simulink model "local_observer_prec"  (R2024b)
settings: Solver=VariableStepAuto  StartTime=0.0  StopTime=20.0  RelTol=1e-3
values from neighbouring files (symbols this model uses):
  A = [0 1; 880.87 0]    [Project.m]    (also in debug_simulink_integration.m; project_multiple_run.m; project_single_run.m)
  B = [0; -9.9453]    [Project.m]    (also in debug_simulink_integration.m; find_hurwitz_F.m = c * eye(n); project_multiple_run.m; project_single_run.m)
  C = [708.27 0]    [Project.m]    (also in debug_simulink_integration.m; project_multiple_run.m; project_single_run.m)
  c = cmin * 2    [Project.m]    (also in project_multiple_run.m = cmin * c_weights(ic); project_single_run.m = cmin)
  K = R^(-1) * B' *Pc    [Project.m]    (also in find_hurwitz_F.m = lqr(A, B, Q, R); project_multiple_run.m = R^(-1) * B' * Pc; project_single_run.m = R^(-1) * B' * Pc)
undefined symbols (not defined in the file or in its folder): A_adj, G_pinning, K_place
settings Model: Creator=fvero  LastModifiedBy=fabio
settings ConfigComp: CovBoundaryAbsTol=1.0e-5

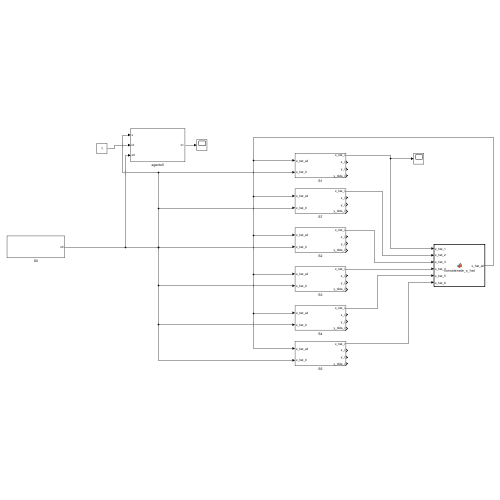
[thumbnail: Simulink's stored preview of the top-level diagram]
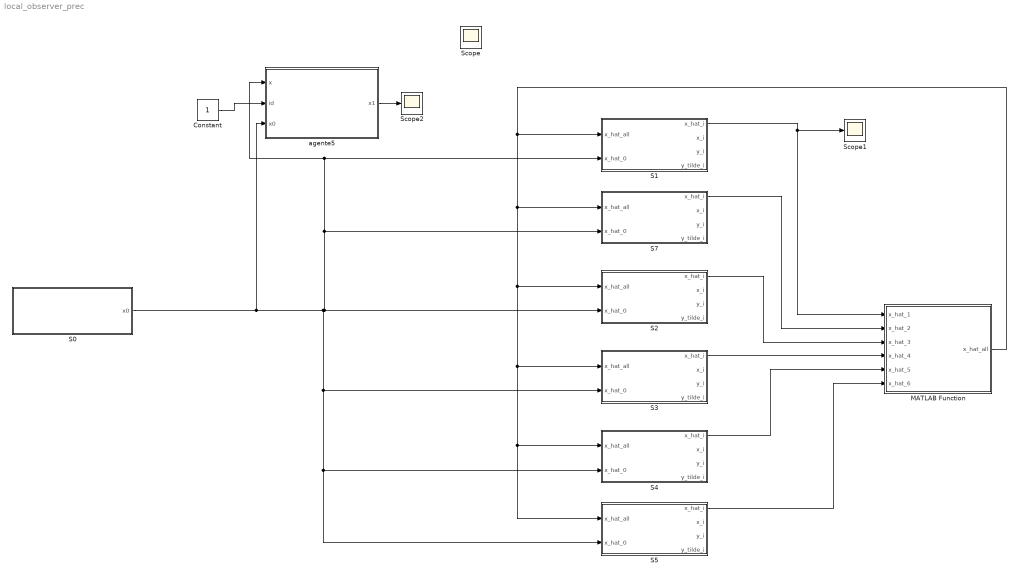
== system local_observer_prec ==
  Constant : Constant
  MATLAB Function : MATLAB Function  TreatAsAtomicUnit=on
  S0 : Subsystem
  S1 : Subsystem
  S2 : Subsystem
  S3 : Subsystem
  S4 : Subsystem
  S5 : Subsystem
  S7 : Subsystem
  Scope1 : Scope
  Scope2 : Scope
  agente5 : Subsystem
  Scope : Scope
  wires:
  S1/1(x_hat_i) -> Scope1/1, MATLAB Function/1(x_hat_1)
  S7/1(x_hat_i) -> MATLAB Function/2(x_hat_2)
  S2/1(x_hat_i) -> MATLAB Function/3(x_hat_3)
  S3/1(x_hat_i) -> MATLAB Function/4(x_hat_4)
  S4/1(x_hat_i) -> MATLAB Function/5(x_hat_5)
  S5/1(x_hat_i) -> MATLAB Function/6(x_hat_6)
  MATLAB Function/1(x_hat_all) -> S7/1(x_hat_all), S2/1(x_hat_all), S3/1(x_hat_all), S5/1(x_hat_all), S4/1(x_hat_all), S1/1(x_hat_all)
  S0/1(x0) -> agente5/3(x0), S3/2(x_hat_0), S5/2(x_hat_0), S4/2(x_hat_0), S2/2(x_hat_0), S7/2(x_hat_0), agente5/1(x), S1/2(x_hat_0)
  Constant/1 -> agente5/2(id)
  agente5/1(x1) -> Scope2/1

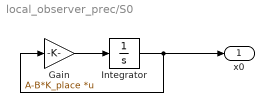
== system local_observer_prec/S0 ==
  Gain : Gain  Gain=A-B*K_place  Multiplication=Matrix(K*u) (u vector)
  Integrator : Integrator  InitialCondition=[10 0]
  x0 : Outport
  wires:
  Gain/1 -> Integrator/1
  Integrator/1 -> x0/1, Gain/1

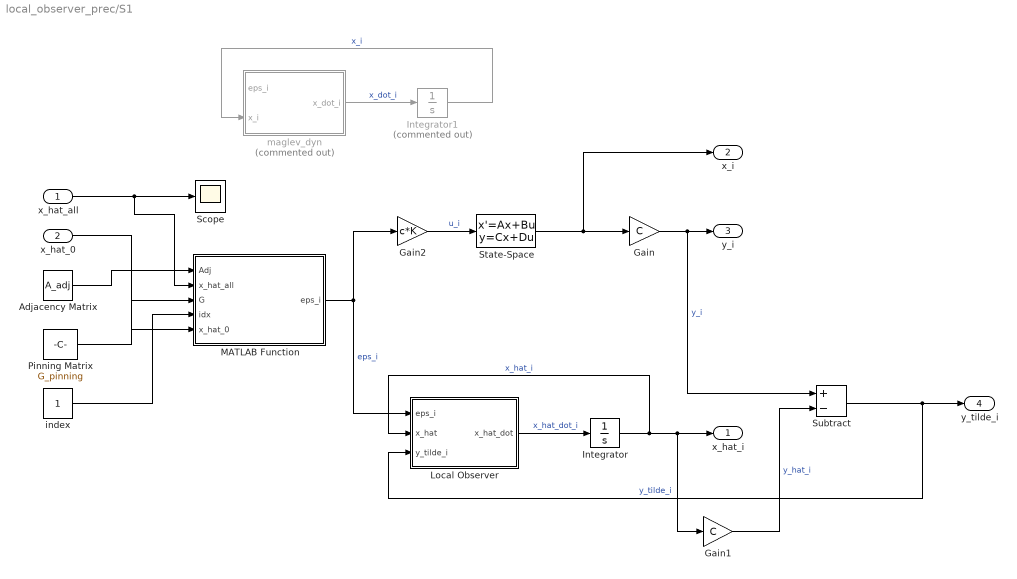
== system local_observer_prec/S1 ==
  x_hat_all : Inport
  x_hat_0 : Inport  Port=2
  "Adjacency Matrix " : Constant  Value=A_adj
  Gain : Gain  Gain=C
  Gain1 : Gain  Gain=C
  Gain2 : Gain  Gain=c*K
  Integrator : Integrator
  Integrator1 : Integrator  Commented=on
  Local Observer : MATLAB Function  TreatAsAtomicUnit=on
  MATLAB Function : MATLAB Function  TreatAsAtomicUnit=on
  Pinning Matrix : Constant  Value=G_pinning
  Scope : Scope
  State-Space : StateSpace  InitialCondition=0
  Subtract : Sum  Inputs=+-
  index : Constant
  maglev_dyn : MATLAB Function  Commented=on  TreatAsAtomicUnit=on
  x_hat_i : Outport
  x_i : Outport  Port=2
  y_i : Outport  Port=3
  y_tilde_i : Outport  Port=4
  wires:
  Local Observer/1(x_hat_dot) -> Integrator/1  "x_hat_dot_i"
  Integrator/1 -> Local Observer/2(x_hat), Gain1/1, x_hat_i/1  "x_hat_i"
  maglev_dyn/1(x_dot_i) -> Integrator1/1  "x_dot_i"
  Integrator1/1 -> maglev_dyn/2(x_i)  "x_i"
  Gain/1 -> Subtract/1, y_i/1  "y_i"
  MATLAB Function/1(eps_i) -> Gain2/1, Local Observer/1(eps_i)  "eps_i"
  Gain2/1 -> State-Space/1  "u_i"
  State-Space/1 -> Gain/1, x_i/1
  x_hat_all/1 -> MATLAB Function/2(x_hat_all), Scope/1
  x_hat_0/1 -> MATLAB Function/5(x_hat_0)
  Pinning Matrix/1 -> MATLAB Function/3(G)
  index/1 -> MATLAB Function/4(idx)
  "Adjacency Matrix "/1 -> MATLAB Function/1(Adj)
  Gain1/1 -> Subtract/2  "y_hat_i"
  Subtract/1 -> Local Observer/3(y_tilde_i), y_tilde_i/1  "y_tilde_i"

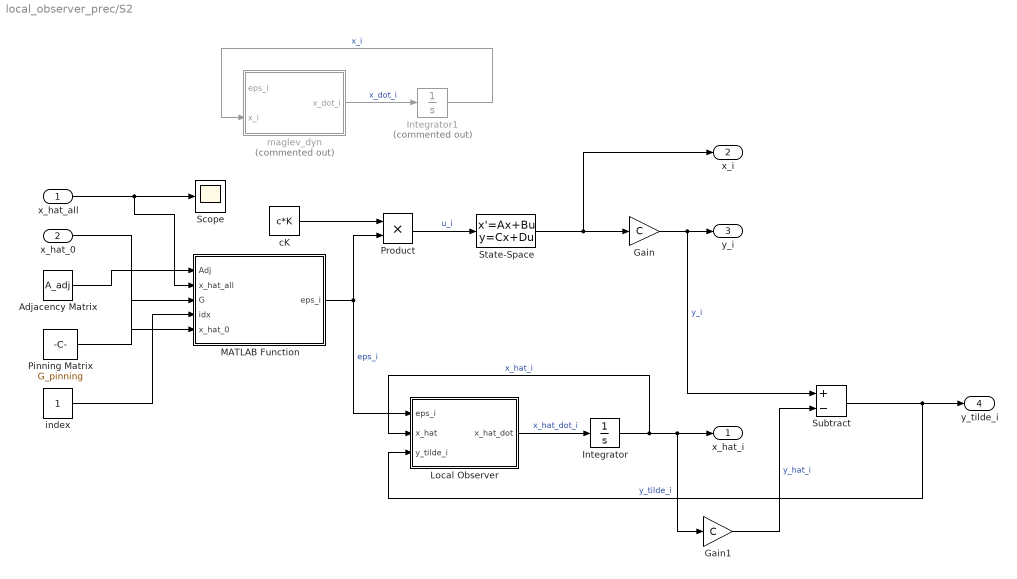
== system local_observer_prec/S2 ==
  x_hat_all : Inport
  x_hat_0 : Inport  Port=2
  "Adjacency Matrix " : Constant  Value=A_adj
  Gain : Gain  Gain=C
  Gain1 : Gain  Gain=C
  Integrator : Integrator
  Integrator1 : Integrator  Commented=on
  Local Observer : MATLAB Function  TreatAsAtomicUnit=on
  MATLAB Function : MATLAB Function  TreatAsAtomicUnit=on
  Pinning Matrix : Constant  Value=G_pinning
  Product : Product
  Scope : Scope
  State-Space : StateSpace  InitialCondition=0
  Subtract : Sum  Inputs=+-
  cK : Constant  Value=c*K
  index : Constant
  maglev_dyn : MATLAB Function  Commented=on  TreatAsAtomicUnit=on
  x_hat_i : Outport
  x_i : Outport  Port=2
  y_i : Outport  Port=3
  y_tilde_i : Outport  Port=4
  wires:
  Local Observer/1(x_hat_dot) -> Integrator/1  "x_hat_dot_i"
  Integrator/1 -> Local Observer/2(x_hat), Gain1/1, x_hat_i/1  "x_hat_i"
  maglev_dyn/1(x_dot_i) -> Integrator1/1  "x_dot_i"
  Integrator1/1 -> maglev_dyn/2(x_i)  "x_i"
  Gain/1 -> Subtract/1, y_i/1  "y_i"
  MATLAB Function/1(eps_i) -> Product/2, Local Observer/1(eps_i)  "eps_i"
  cK/1 -> Product/1
  Product/1 -> State-Space/1  "u_i"
  State-Space/1 -> Gain/1, x_i/1
  x_hat_all/1 -> MATLAB Function/2(x_hat_all), Scope/1
  x_hat_0/1 -> MATLAB Function/5(x_hat_0)
  Pinning Matrix/1 -> MATLAB Function/3(G)
  index/1 -> MATLAB Function/4(idx)
  "Adjacency Matrix "/1 -> MATLAB Function/1(Adj)
  Gain1/1 -> Subtract/2  "y_hat_i"
  Subtract/1 -> Local Observer/3(y_tilde_i), y_tilde_i/1  "y_tilde_i"

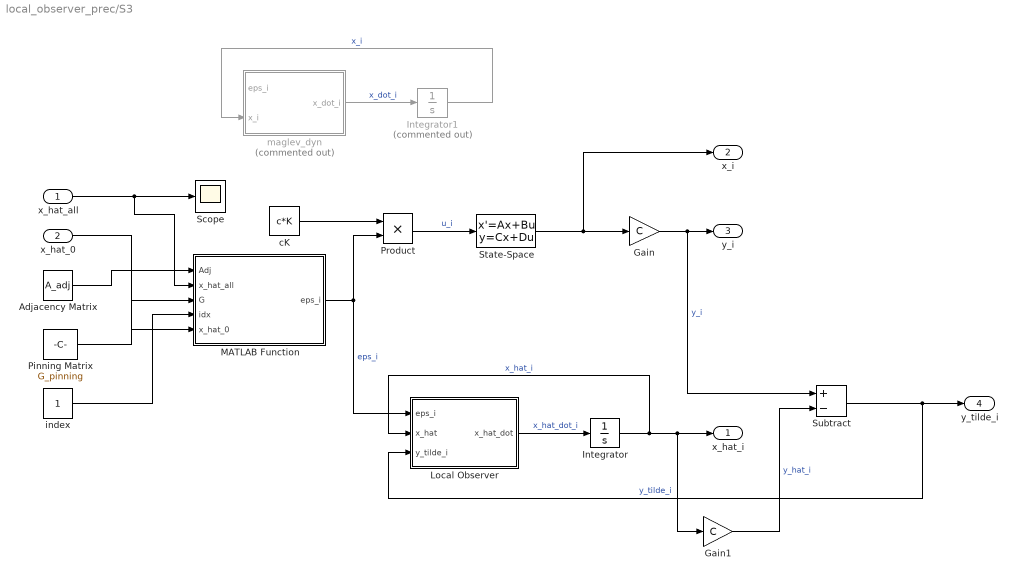
== system local_observer_prec/S3 ==
  x_hat_all : Inport
  x_hat_0 : Inport  Port=2
  "Adjacency Matrix " : Constant  Value=A_adj
  Gain : Gain  Gain=C
  Gain1 : Gain  Gain=C
  Integrator : Integrator
  Integrator1 : Integrator  Commented=on
  Local Observer : MATLAB Function  TreatAsAtomicUnit=on
  MATLAB Function : MATLAB Function  TreatAsAtomicUnit=on
  Pinning Matrix : Constant  Value=G_pinning
  Product : Product
  Scope : Scope
  State-Space : StateSpace  InitialCondition=0
  Subtract : Sum  Inputs=+-
  cK : Constant  Value=c*K
  index : Constant
  maglev_dyn : MATLAB Function  Commented=on  TreatAsAtomicUnit=on
  x_hat_i : Outport
  x_i : Outport  Port=2
  y_i : Outport  Port=3
  y_tilde_i : Outport  Port=4
  wires:
  Local Observer/1(x_hat_dot) -> Integrator/1  "x_hat_dot_i"
  Integrator/1 -> Local Observer/2(x_hat), Gain1/1, x_hat_i/1  "x_hat_i"
  maglev_dyn/1(x_dot_i) -> Integrator1/1  "x_dot_i"
  Integrator1/1 -> maglev_dyn/2(x_i)  "x_i"
  Gain/1 -> Subtract/1, y_i/1  "y_i"
  MATLAB Function/1(eps_i) -> Product/2, Local Observer/1(eps_i)  "eps_i"
  cK/1 -> Product/1
  Product/1 -> State-Space/1  "u_i"
  State-Space/1 -> Gain/1, x_i/1
  x_hat_all/1 -> MATLAB Function/2(x_hat_all), Scope/1
  x_hat_0/1 -> MATLAB Function/5(x_hat_0)
  Pinning Matrix/1 -> MATLAB Function/3(G)
  index/1 -> MATLAB Function/4(idx)
  "Adjacency Matrix "/1 -> MATLAB Function/1(Adj)
  Gain1/1 -> Subtract/2  "y_hat_i"
  Subtract/1 -> Local Observer/3(y_tilde_i), y_tilde_i/1  "y_tilde_i"

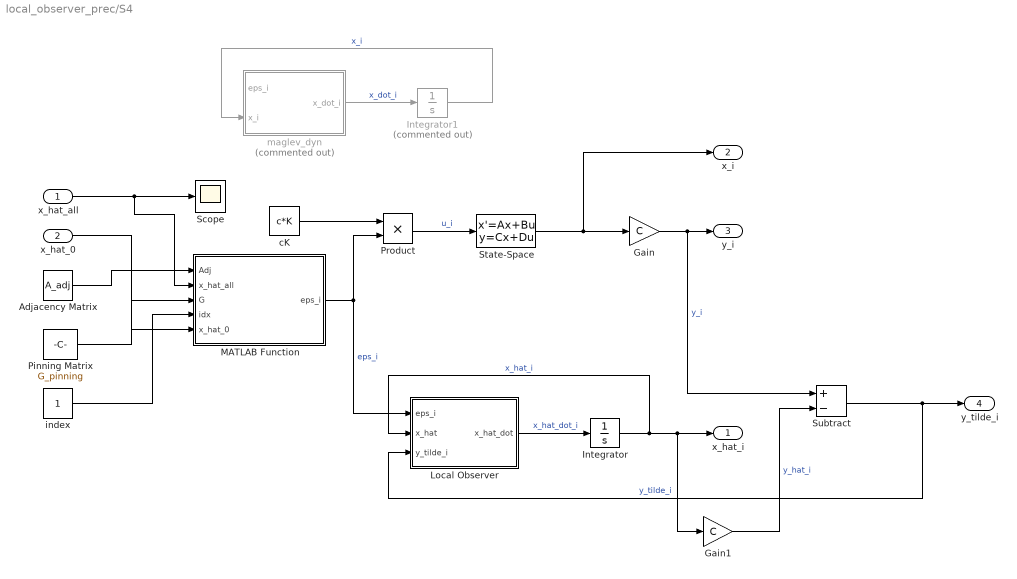
== system local_observer_prec/S4 ==
  x_hat_all : Inport
  x_hat_0 : Inport  Port=2
  "Adjacency Matrix " : Constant  Value=A_adj
  Gain : Gain  Gain=C
  Gain1 : Gain  Gain=C
  Integrator : Integrator
  Integrator1 : Integrator  Commented=on
  Local Observer : MATLAB Function  TreatAsAtomicUnit=on
  MATLAB Function : MATLAB Function  TreatAsAtomicUnit=on
  Pinning Matrix : Constant  Value=G_pinning
  Product : Product
  Scope : Scope
  State-Space : StateSpace  InitialCondition=0
  Subtract : Sum  Inputs=+-
  cK : Constant  Value=c*K
  index : Constant
  maglev_dyn : MATLAB Function  Commented=on  TreatAsAtomicUnit=on
  x_hat_i : Outport
  x_i : Outport  Port=2
  y_i : Outport  Port=3
  y_tilde_i : Outport  Port=4
  wires:
  Local Observer/1(x_hat_dot) -> Integrator/1  "x_hat_dot_i"
  Integrator/1 -> Local Observer/2(x_hat), Gain1/1, x_hat_i/1  "x_hat_i"
  maglev_dyn/1(x_dot_i) -> Integrator1/1  "x_dot_i"
  Integrator1/1 -> maglev_dyn/2(x_i)  "x_i"
  Gain/1 -> Subtract/1, y_i/1  "y_i"
  MATLAB Function/1(eps_i) -> Product/2, Local Observer/1(eps_i)  "eps_i"
  cK/1 -> Product/1
  Product/1 -> State-Space/1  "u_i"
  State-Space/1 -> Gain/1, x_i/1
  x_hat_all/1 -> MATLAB Function/2(x_hat_all), Scope/1
  x_hat_0/1 -> MATLAB Function/5(x_hat_0)
  Pinning Matrix/1 -> MATLAB Function/3(G)
  index/1 -> MATLAB Function/4(idx)
  "Adjacency Matrix "/1 -> MATLAB Function/1(Adj)
  Gain1/1 -> Subtract/2  "y_hat_i"
  Subtract/1 -> Local Observer/3(y_tilde_i), y_tilde_i/1  "y_tilde_i"

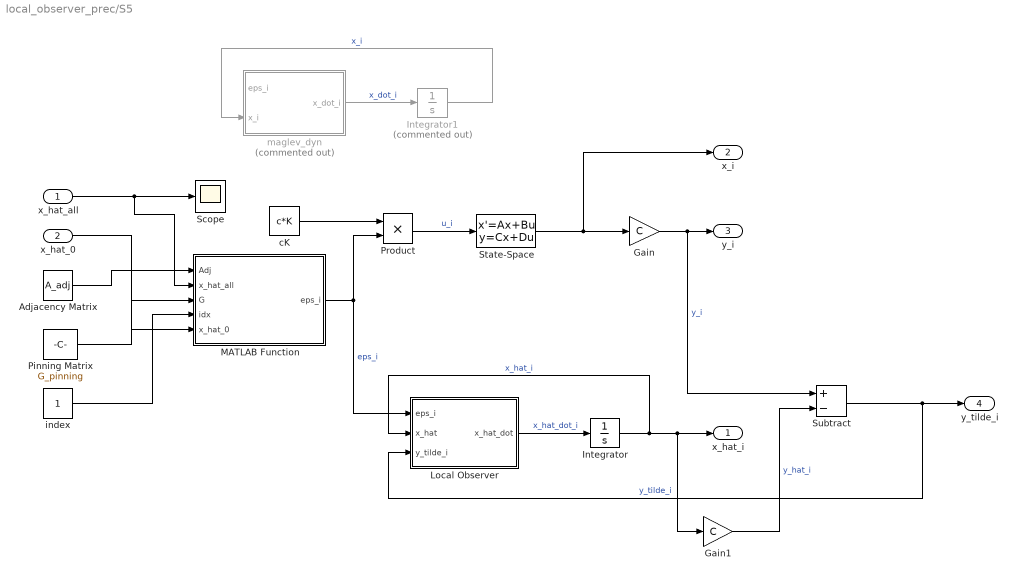
== system local_observer_prec/S5 ==
  x_hat_all : Inport
  x_hat_0 : Inport  Port=2
  "Adjacency Matrix " : Constant  Value=A_adj
  Gain : Gain  Gain=C
  Gain1 : Gain  Gain=C
  Integrator : Integrator
  Integrator1 : Integrator  Commented=on
  Local Observer : MATLAB Function  TreatAsAtomicUnit=on
  MATLAB Function : MATLAB Function  TreatAsAtomicUnit=on
  Pinning Matrix : Constant  Value=G_pinning
  Product : Product
  Scope : Scope
  State-Space : StateSpace  InitialCondition=0
  Subtract : Sum  Inputs=+-
  cK : Constant  Value=c*K
  index : Constant
  maglev_dyn : MATLAB Function  Commented=on  TreatAsAtomicUnit=on
  x_hat_i : Outport
  x_i : Outport  Port=2
  y_i : Outport  Port=3
  y_tilde_i : Outport  Port=4
  wires:
  Local Observer/1(x_hat_dot) -> Integrator/1  "x_hat_dot_i"
  Integrator/1 -> Local Observer/2(x_hat), Gain1/1, x_hat_i/1  "x_hat_i"
  maglev_dyn/1(x_dot_i) -> Integrator1/1  "x_dot_i"
  Integrator1/1 -> maglev_dyn/2(x_i)  "x_i"
  Gain/1 -> Subtract/1, y_i/1  "y_i"
  MATLAB Function/1(eps_i) -> Product/2, Local Observer/1(eps_i)  "eps_i"
  cK/1 -> Product/1
  Product/1 -> State-Space/1  "u_i"
  State-Space/1 -> Gain/1, x_i/1
  x_hat_all/1 -> MATLAB Function/2(x_hat_all), Scope/1
  x_hat_0/1 -> MATLAB Function/5(x_hat_0)
  Pinning Matrix/1 -> MATLAB Function/3(G)
  index/1 -> MATLAB Function/4(idx)
  "Adjacency Matrix "/1 -> MATLAB Function/1(Adj)
  Gain1/1 -> Subtract/2  "y_hat_i"
  Subtract/1 -> Local Observer/3(y_tilde_i), y_tilde_i/1  "y_tilde_i"

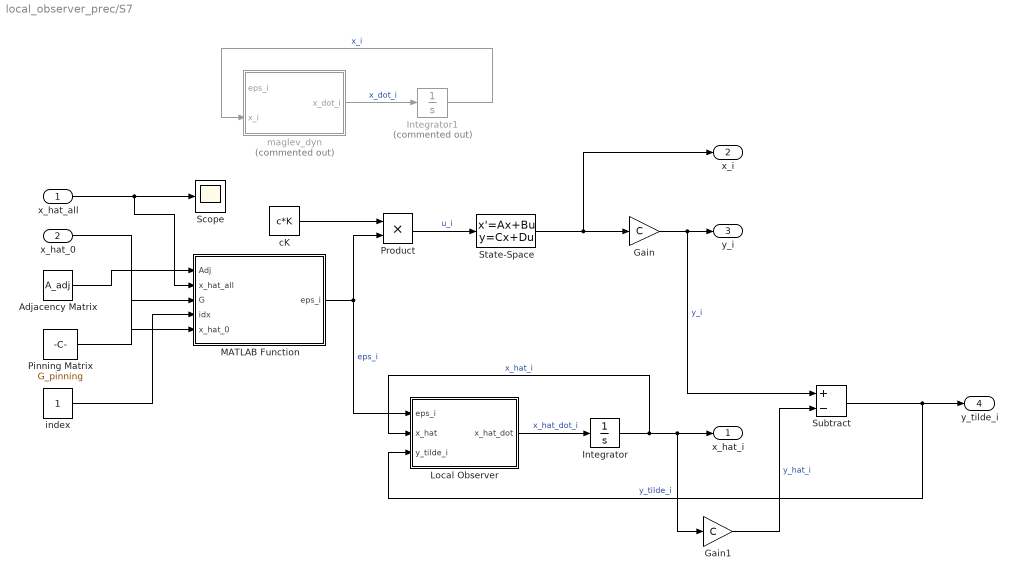
== system local_observer_prec/S7 ==
  x_hat_all : Inport
  x_hat_0 : Inport  Port=2
  "Adjacency Matrix " : Constant  Value=A_adj
  Gain : Gain  Gain=C
  Gain1 : Gain  Gain=C
  Integrator : Integrator
  Integrator1 : Integrator  Commented=on
  Local Observer : MATLAB Function  TreatAsAtomicUnit=on
  MATLAB Function : MATLAB Function  TreatAsAtomicUnit=on
  Pinning Matrix : Constant  Value=G_pinning
  Product : Product
  Scope : Scope
  State-Space : StateSpace  InitialCondition=0
  Subtract : Sum  Inputs=+-
  cK : Constant  Value=c*K
  index : Constant
  maglev_dyn : MATLAB Function  Commented=on  TreatAsAtomicUnit=on
  x_hat_i : Outport
  x_i : Outport  Port=2
  y_i : Outport  Port=3
  y_tilde_i : Outport  Port=4
  wires:
  Local Observer/1(x_hat_dot) -> Integrator/1  "x_hat_dot_i"
  Integrator/1 -> Local Observer/2(x_hat), Gain1/1, x_hat_i/1  "x_hat_i"
  maglev_dyn/1(x_dot_i) -> Integrator1/1  "x_dot_i"
  Integrator1/1 -> maglev_dyn/2(x_i)  "x_i"
  Gain/1 -> Subtract/1, y_i/1  "y_i"
  MATLAB Function/1(eps_i) -> Product/2, Local Observer/1(eps_i)  "eps_i"
  cK/1 -> Product/1
  Product/1 -> State-Space/1  "u_i"
  State-Space/1 -> Gain/1, x_i/1
  x_hat_all/1 -> MATLAB Function/2(x_hat_all), Scope/1
  x_hat_0/1 -> MATLAB Function/5(x_hat_0)
  Pinning Matrix/1 -> MATLAB Function/3(G)
  index/1 -> MATLAB Function/4(idx)
  "Adjacency Matrix "/1 -> MATLAB Function/1(Adj)
  Gain1/1 -> Subtract/2  "y_hat_i"
  Subtract/1 -> Local Observer/3(y_tilde_i), y_tilde_i/1  "y_tilde_i"

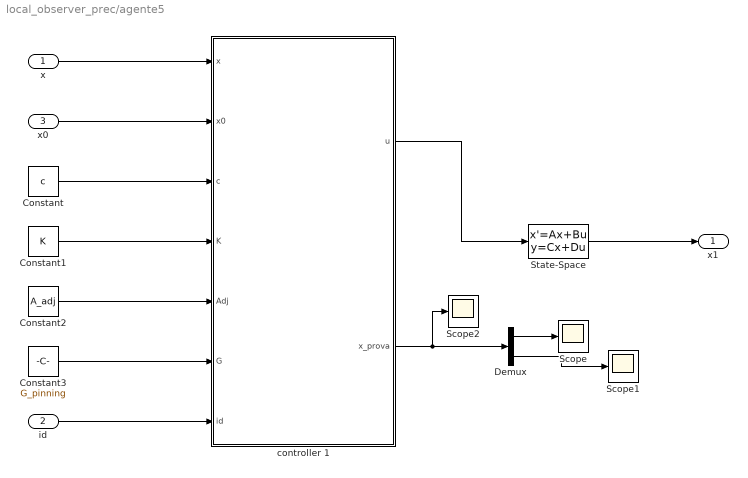
== system local_observer_prec/agente5 ==
  x : Inport
  id : Inport  Port=2
  x0 : Inport  Port=3
  Constant : Constant  Value=c
  Constant1 : Constant  Value=K  VectorParams1D=off
  Constant2 : Constant  Value=A_adj
  Constant3 : Constant  Value=G_pinning
  Demux : Demux  Outputs=2
  Scope : Scope
  Scope1 : Scope
  Scope2 : Scope
  State-Space : StateSpace  A=A-B*K  B=B  C=eye(2)  D=zeros(2,1)  InitialCondition=0
  controller 1 : MATLAB Function  TreatAsAtomicUnit=on
  x1 : Outport
  wires:
  Demux/2 -> Scope1/1
  Demux/1 -> Scope/1
  x0/1 -> controller 1/2(x0)
  Constant2/1 -> controller 1/5(Adj)
  Constant1/1 -> controller 1/4(K)
  id/1 -> controller 1/7(id)
  Constant3/1 -> controller 1/6(G)
  State-Space/1 -> x1/1
  controller 1/1(u) -> State-Space/1
  controller 1/2(x_prova) -> Scope2/1, Demux/1
  x/1 -> controller 1/1(x)
  Constant/1 -> controller 1/3(c)

== matlab function local_observer_prec/S4/MATLAB Function ==
  data: Adj input; eps_i output; x_hat_all input; G input; idx input; x_hat_0 input
function eps_i = compute_eps(Adj, x_hat_all, G, idx, x_hat_0)

Adj_i = Adj(idx, :);
g_i = G(idx, idx);

x_hat_i = x_hat_all(idx, :)'; %2*1

diff = g_i * (x_hat_0 - x_hat_i); 

eps_i = zeros(2,1); 

for j = 1:6
    eps_i = eps_i + Adj_i(j)*(x_hat_all(j,:)' - x_hat_i) + diff; 
end 

end

== matlab function local_observer_prec/S4/maglev_dyn ==
  data: eps_i input; x_dot_i output; x_i input
function x_dot_i = maglev_dyn(eps_i, x_i)
    
    u_i = c*K*eps_i;
    x_dot_i = A * x_i + B*u_i;

end

== matlab function local_observer_prec/S5/Local Observer ==
  data: eps_i input; x_hat_dot output; x_hat input; y_tilde_i input
function x_hat_dot = observer(eps_i, x_hat, y_tilde_i)
    
    u_i = c*K*eps_i;
    x_hat_dot = A * x_hat + B*u_i - c*F*y_tilde_i;

end

== matlab function local_observer_prec/S5/MATLAB Function ==
  data: Adj input; eps_i output; x_hat_all input; G input; idx input; x_hat_0 input
function eps_i = compute_eps(Adj, x_hat_all, G, idx, x_hat_0)

Adj_i = Adj(idx, :);
g_i = G(idx, idx);

x_hat_i = x_hat_all(idx, :)'; %2*1

diff = g_i * (x_hat_0 - x_hat_i); 

eps_i = zeros(2,1); 

for j = 1:6
    eps_i = eps_i + Adj_i(j)*(x_hat_all(j,:)' - x_hat_i) + diff; 
end 

end

== matlab function local_observer_prec/S1/Local Observer ==
  data: eps_i input; x_hat_dot output; x_hat input; y_tilde_i input
function x_hat_dot = observer(eps_i, x_hat, y_tilde_i)
    
    u_i = c*K*eps_i;
    x_hat_dot = A * x_hat + B*u_i - c*F*y_tilde_i;

end

== matlab function local_observer_prec/S5/maglev_dyn ==
  data: eps_i input; x_dot_i output; x_i input
function x_dot_i = maglev_dyn(eps_i, x_i)
    
    u_i = c*K*eps_i;
    x_dot_i = A * x_i + B*u_i;

end

== matlab function local_observer_prec/agente5/controller 1 ==
  data: x input; x0 input; u output; c input; K input; Adj input; G input; id input; x_prova output
function [u,x_prova]= controller(x,x0,c,K,Adj,G,id)


pairs = x;

error = zeros(2,1);

for j = 1:6
    error = error + Adj(id,j)*(pairs(j,:)'-pairs(id,:)')+G(id)*(x0 - pairs(id,:)');
end

x_prova = pairs(id,:)';

u=c*K*error;

== matlab function local_observer_prec/MATLAB Function ==
  data: x_hat_1 input; x_hat_all output; x_hat_2 input; x_hat_3 input; x_hat_4 input; x_hat_5 input; x_hat_6 input
function x_hat_all = concatenate_x_hat(x_hat_1, x_hat_2, x_hat_3, x_hat_4, x_hat_5, x_hat_6)

x_hat_all = [x_hat_1'; x_hat_2'; x_hat_3'; x_hat_4'; x_hat_5'; x_hat_6'];

end

== matlab function local_observer_prec/S7/Local Observer ==
  data: eps_i input; x_hat_dot output; x_hat input; y_tilde_i input
function x_hat_dot = observer(eps_i, x_hat, y_tilde_i)
    
    u_i = c*K*eps_i;
    x_hat_dot = A * x_hat + B*u_i - c*F*y_tilde_i;

end

== matlab function local_observer_prec/S7/MATLAB Function ==
  data: Adj input; eps_i output; x_hat_all input; G input; idx input; x_hat_0 input
function eps_i = compute_eps(Adj, x_hat_all, G, idx, x_hat_0)

Adj_i = Adj(idx, :);
g_i = G(idx, idx);

x_hat_i = x_hat_all(idx, :)'; %2*1

diff = g_i * (x_hat_0 - x_hat_i); 

eps_i = zeros(2,1); 

for j = 1:6
    eps_i = eps_i + Adj_i(j)*(x_hat_all(j,:)' - x_hat_i) + diff; 
end 

end

== matlab function local_observer_prec/S7/maglev_dyn ==
  data: eps_i input; x_dot_i output; x_i input
function x_dot_i = maglev_dyn(eps_i, x_i)
    
    u_i = c*K*eps_i;
    x_dot_i = A * x_i + B*u_i;

end

== matlab function local_observer_prec/S1/MATLAB Function ==
  data: Adj input; eps_i output; x_hat_all input; G input; idx input; x_hat_0 input
function eps_i = compute_eps(Adj, x_hat_all, G, idx, x_hat_0)

Adj_i = Adj(idx, :);
g_i = G(idx, idx);

x_hat_i = x_hat_all(idx, :)'; %2*1

diff = g_i * (x_hat_0 - x_hat_i)'; 

eps_i = zeros(2,1); 

for j = 1:6
    eps_i = eps_i + Adj_i(j)*(x_hat_all(j,:)' - x_hat_i) + diff; 
end 

end

== matlab function local_observer_prec/S1/maglev_dyn ==
  data: eps_i input; x_dot_i output; x_i input
function x_dot_i = maglev_dyn(eps_i, x_i)
    
    u_i = c*K*eps_i;
    x_dot_i = A * x_i + B*u_i;

end

== matlab function local_observer_prec/S2/Local Observer ==
  data: eps_i input; x_hat_dot output; x_hat input; y_tilde_i input
function x_hat_dot = observer(eps_i, x_hat, y_tilde_i)
    
    u_i = c*K*eps_i;
    x_hat_dot = A * x_hat + B*u_i - c*F*y_tilde_i;

end

== matlab function local_observer_prec/S2/MATLAB Function ==
  data: Adj input; eps_i output; x_hat_all input; G input; idx input; x_hat_0 input
function eps_i = compute_eps(Adj, x_hat_all, G, idx, x_hat_0)

Adj_i = Adj(idx, :);
g_i = G(idx, idx);

x_hat_i = x_hat_all(idx, :)'; %2*1

diff = g_i * (x_hat_0 - x_hat_i); 

eps_i = zeros(2,1); 

for j = 1:6
    eps_i = eps_i + Adj_i(j)*(x_hat_all(j,:)' - x_hat_i) + diff; 
end 

end

== matlab function local_observer_prec/S2/maglev_dyn ==
  data: eps_i input; x_dot_i output; x_i input
function x_dot_i = maglev_dyn(eps_i, x_i)
    
    u_i = c*K*eps_i;
    x_dot_i = A * x_i + B*u_i;

end

== matlab function local_observer_prec/S3/Local Observer ==
  data: eps_i input; x_hat_dot output; x_hat input; y_tilde_i input
function x_hat_dot = observer(eps_i, x_hat, y_tilde_i)
    
    u_i = c*K*eps_i;
    x_hat_dot = A * x_hat + B*u_i - c*F*y_tilde_i;

end

== matlab function local_observer_prec/S3/MATLAB Function ==
  data: Adj input; eps_i output; x_hat_all input; G input; idx input; x_hat_0 input
function eps_i = compute_eps(Adj, x_hat_all, G, idx, x_hat_0)

Adj_i = Adj(idx, :);
g_i = G(idx, idx);

x_hat_i = x_hat_all(idx, :)'; %2*1

diff = g_i * (x_hat_0 - x_hat_i); 

eps_i = zeros(2,1); 

for j = 1:6
    eps_i = eps_i + Adj_i(j)*(x_hat_all(j,:)' - x_hat_i) + diff; 
end 

end

== matlab function local_observer_prec/S3/maglev_dyn ==
  data: eps_i input; x_dot_i output; x_i input
function x_dot_i = maglev_dyn(eps_i, x_i)
    
    u_i = c*K*eps_i;
    x_dot_i = A * x_i + B*u_i;

end

== matlab function local_observer_prec/S4/Local Observer ==
  data: eps_i input; x_hat_dot output; x_hat input; y_tilde_i input
function x_hat_dot = observer(eps_i, x_hat, y_tilde_i)
    
    u_i = c*K*eps_i;
    x_hat_dot = A * x_hat + B*u_i - c*F*y_tilde_i;

end
